simulink model "relay_sim"  (R2013a)
settings: Solver=ode3  StartTime=0.0  StopTime=20  FixedStep=0.1  RelTol=1e-3
values from neighbouring files (symbols this model uses):
  a = 1    [relay_param.m]
  a_offset = 0    [relay_param.m]
  h = h+0.4    (= 0.4)    [relay_param.m]
  h_offset = 0    [relay_param.m]
settings Model: Creator=Thomas  LastModifiedBy=Thomas

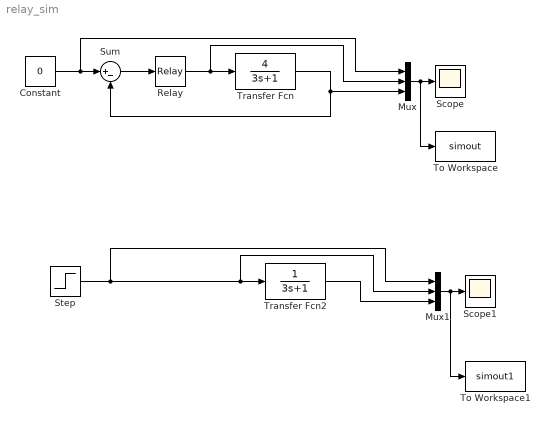
== system relay_sim ==
  Constant : Constant  Value=0
  Mux : Mux  Inputs=3
  Mux1 : Mux  Inputs=3
  Relay : Relay  OnSwitchValue=+h/2+h_offset  OffSwitchValue=-h/2+h_offset  OnOutputValue=a+a_offset  OffOutputValue=-a+a_offset
  Scope : Scope
      settings: TimeRange=10  YMin=-1  YMax=1
  Scope1 : Scope
      settings: TimeRange=20  YMin=-1  YMax=1
  Step : Step  Time=0  SampleTime=0
  Sum : Sum  Inputs=|+-
  To Workspace : ToWorkspace  VariableName=simout  SampleTime=-1
  To Workspace1 : ToWorkspace  VariableName=simout1  SampleTime=-1
  Transfer Fcn : TransferFcn  Numerator=[4]  Denominator=[3 1]
  Transfer Fcn2 : TransferFcn  Denominator=[3 1]
  wires:
  Constant/1 -> Mux/1, Sum/1
  Sum/1 -> Relay/1
  Relay/1 -> Mux/2, Transfer Fcn/1
  Transfer Fcn/1 -> Mux/3, Sum/2
  Mux/1 -> To Workspace/1, Scope/1
  Step/1 -> Mux1/2, Transfer Fcn2/1, Mux1/1
  Transfer Fcn2/1 -> Mux1/3
  Mux1/1 -> To Workspace1/1, Scope1/1
